simulink model "pathtest"  (Simulink 7.6)
settings: Solver=ode45  StartTime=0.0  StopTime=1  RelTol=1e-3
undefined symbols (not defined in the file): jet, Rec, SDTV
libraries: vipconversions x1, vipsrcs x1, vipsnks x1
settings Model: Creator=auvt  LastModifiedBy=auvt

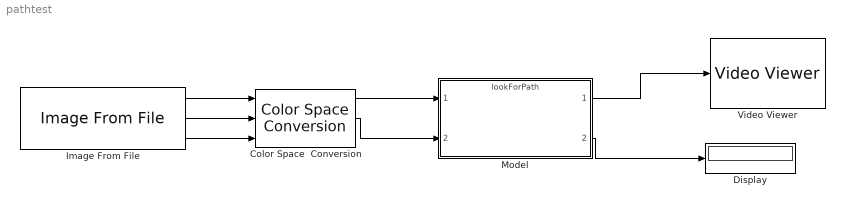
== system pathtest ==
  Color Space  Conversion : vipconversions/Color Space  Conversion  conversion=Obsolete  conversionActive=R'G'B' to HSV  wp_str=D65  rec=Rec. 601 (SDTV)  sys=1125/60/2:1  imagePorts=Separate color signals
  Display : Display
  Image From File : vipsrcs/Image From File  Tag=vipblks_nd  DialogController=vipDDGCreate  DialogControllerArgs=DataTag0  SystemSampleTime=-1  FileName=/home/auvt/auvc/tests/paths/control.png  imagePorts=Separate color signals  Ts=inf  ImageDataType=double  Signed=on  WordLength=16  sdImageDataType=uint(8)  FractionLengthMode=User-defined  FractionLength=15  OutPortLabels=R|G|B
  Model : ModelReference  ModelNameDialog=lookForPath  SimulationMode=Accelerator  ModelReferenceVersion=1.2  CopyOfModelName=lookForPath
  Video Viewer : vipsnks/Video Viewer  DialogControllerArgs=DataTag2  inputType=Obsolete7b  imagePorts=One multidimensional signal  useColorMap=off  colormapValue=jet(256)  specRange=off  minInputVal=0  maxInputVal=255  FigPos=[2350 707 643 501]  AxisZoom=on  trueSizedOnce=off  OpenAtMdlStart=on
  wires:
  Image From File/1 -> Color Space  Conversion/1
  Color Space  Conversion/1 -> Model/1
  Color Space  Conversion/2 -> Model/2
  Model/1 -> Video Viewer/1
  Model/2 -> Display/1
  Image From File/2 -> Color Space  Conversion/2
  Image From File/3 -> Color Space  Conversion/3
